simulink model "Masse_MultirotorSimHinf"  (R2018b)
settings: Solver=VariableStepAuto  StartTime=0.0  StopTime=Simulation.T_END  MaxStep=Simulation.TS_MAX  RelTol=1e-3  EnableMultiTasking=on
PreLoadFcn:
  | % InitializeParameters;
undefined symbols (not defined in the file): Aero, armed, ctrl_state, INIT_PARAM_VECTOR, Initial, K_i, K_p, Motor, mpc_att_sp, mpc_ctrl_state, mpc_manual, mpc_pos_sp_triplet, mpc_vehicle_land_detected, mpc_vehicle_status, Simulation, SOF1, SOF2, Uav, Upsilon, v_att_sp, v_control_mode
libraries: simulink_extras x9, simulink x6, dspstat3 x1, Px4Library x1
(part 3 of 11)

== system Masse_MultirotorSimHinf/Quadrotor Quaternion Model/Compute S Matrix2 ==
  quaternion : Inport
  MATLAB Function : MATLAB Function  TreatAsAtomicUnit=on
  rotationMatrix : Outport
  wires:
  quaternion/1 -> MATLAB Function/1(q)
  MATLAB Function/1(S) -> rotationMatrix/1

== system Masse_MultirotorSimHinf/Quadrotor Quaternion Model/Normalise Quaternion ==
  quaternion : Inport
  MATLAB Function : MATLAB Function  TreatAsAtomicUnit=on
  normalised : Outport
  wires:
  quaternion/1 -> MATLAB Function/1(q)
  MATLAB Function/1(qOut) -> normalised/1

== system Masse_MultirotorSimHinf/Quadrotor Quaternion Model/Quaternion to Euler Angles ==
  quaternion : Inport
  MATLAB Function : MATLAB Function  TreatAsAtomicUnit=on
  euler : Outport
  wires:
  quaternion/1 -> MATLAB Function/1(quat)
  MATLAB Function/1(eul) -> euler/1

== system Masse_MultirotorSimHinf/Quadrotor Quaternion Model/Quaternion to Rotation Matrix ==
  quaternion : Inport
  MATLAB Function : MATLAB Function  TreatAsAtomicUnit=on
  rotationMatrix : Outport
  wires:
  MATLAB Function/1(R) -> rotationMatrix/1
  quaternion/1 -> MATLAB Function/1(q)

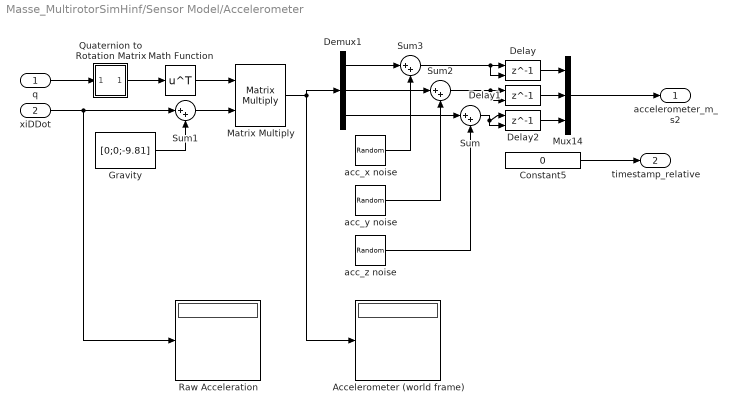
== system Masse_MultirotorSimHinf/Sensor Model/Accelerometer ==
  q : Inport
  xiDDot : Inport  Port=2  Unit=m/s^2
  Accelerometer (world frame) : Display
  Constant5 : Constant  Value=0
  Delay : Delay  DelayLength=1  InitialConditionSource=Input port  SampleTime=1/400
      settings: InputPortMap=u0,p4
  Delay1 : Delay  DelayLength=1  InitialConditionSource=Input port  SampleTime=1/400
      settings: InputPortMap=u0,p4
  Delay2 : Delay  DelayLength=1  InitialConditionSource=Input port  SampleTime=1/400
      settings: InputPortMap=u0,p4
  Demux1 : Demux  Outputs=3
  Gravity : Constant  Value=[0;0;-9.81]
  Math Function : Math  Operator=transpose  SaturateOnIntegerOverflow=on
  Matrix Multiply : Product  Multiplication=Matrix(*)
  Mux14 : Mux  Inputs=3
  Quaternion to Rotation Matrix : Subsystem  AncestorBlock=QuaternionLibrary/Quaternion to Rotation Matrix
      mask help: Convert an orientation quaternion to an orthogonal transformation matrix
      mask Help:
      | Convert an orientation quaternion
      | [q1 q2 q3 q4]
      | where:
      | - q1 is the rotation in radians
      | - [q2 q3 q4] is the vector around which the rotation is performed)
      | to an orthogonal transformation matrix
      | Based on code from the PX4 firmware: https://github.com/PX4/Firmware
      mask Display: disp('Q2R')
  Raw Acceleration : Display
  Sum{,1..3} (4 alike) : Sum  Inputs=|++
  acc_x noise : RandomNumber  Variance=0.012^2  SampleTime=1/400
  acc_y noise : RandomNumber  Variance=0.012^2  SampleTime=1/400
  acc_z noise : RandomNumber  Variance=0.02^2  SampleTime=1/400
  accelerometer_m_s2 : Outport  Unit=m/s^2  SampleTime=1/400
  timestamp_relative : Outport  Port=2  Unit=µs  SampleTime=1/400
  wires:
  Quaternion to Rotation Matrix/1(rotationMatrix) -> Math Function/1
  Math Function/1 -> Matrix Multiply/1
  Matrix Multiply/1 -> Accelerometer (world frame)/1, Demux1/1
  Gravity/1 -> Sum1/2
  Sum1/1 -> Matrix Multiply/2
  Mux14/1 -> accelerometer_m_s2/1
  xiDDot/1 -> Raw Acceleration/1, Sum1/1
  q/1 -> Quaternion to Rotation Matrix/1(quaternion)
  Constant5/1 -> timestamp_relative/1
  Demux1/1 -> Sum3/1
  Demux1/2 -> Sum2/1
  Demux1/3 -> Sum/1
  Sum/1 -> Delay2/2, Delay2/1
  acc_z noise/1 -> Sum/2
  Sum2/1 -> Delay1/2, Delay1/1
  Sum3/1 -> Delay/2, Delay/1
  acc_y noise/1 -> Sum2/2
  acc_x noise/1 -> Sum3/2
  Delay/1 -> Mux14/1
  Delay1/1 -> Mux14/2
  Delay2/1 -> Mux14/3

== system Masse_MultirotorSimHinf/Sensor Model/Barometer ==
  xi : Inport  Unit=m
  timestamp : Inport  Port=2  Unit=µs
  Add : Sum  Inputs=+-
  Scope : Scope
  Select altitude : Selector  InputPortWidth=3  IndexOptions=Index vector (dialog)  Indices=3  OutputSizes=1
  Sum : Sum  Inputs=|++
  To 400 Hz : RateTransition  Deterministic=off  OutPortSampleTime=1/250
  To 400 Hz1 : RateTransition  OutPortSampleTime=1/400
  To 50 Hz : RateTransition  OutPortSampleTime=1/50
  To 50 Hz1 : RateTransition  OutPortSampleTime=1/50
  barro noise : RandomNumber  Variance=1/3^2  SampleTime=0.01
  baro_alt_meter : Outport  Unit=m  SampleTime=1/400
  timestamp_relative : Outport  Port=2  Unit=µs
  wires:
  barro noise/1 -> Sum/2
  Sum/1 -> To 50 Hz1/1
  xi/1 -> Select altitude/1
  Select altitude/1 -> Sum/1
  Add/1 -> timestamp_relative/1, Scope/1
  To 400 Hz1/1 -> Add/2
  To 50 Hz/1 -> To 400 Hz/1
  To 400 Hz/1 -> Add/1
  timestamp/1 -> To 50 Hz/1, To 400 Hz1/1
  To 50 Hz1/1 -> baro_alt_meter/1

== system Masse_MultirotorSimHinf/Sensor Model/Global reprojection ==
  x : Inport
  y : Inport  Port=2
  map_projection_reproject : MATLAB Function  TreatAsAtomicUnit=on
  lat : Outport
  lon : Outport  Port=2
  wires:
  y/1 -> map_projection_reproject/2(y)
  map_projection_reproject/2(lon) -> lon/1
  x/1 -> map_projection_reproject/1(x)
  map_projection_reproject/1(lat) -> lat/1

== system Masse_MultirotorSimHinf/Sensor Model/Gyroscope ==
  nuBody : Inport  Unit=rad/s
  Bias : Constant  Commented=on  Value=[0.0001;0.0001;0.0001]
  Delay1 : Delay  DelayLength=1  InitialConditionSource=Input port  SampleTime=1/400
      settings: InputPortMap=u0,p4
  Delay2 : Delay  DelayLength=1  InitialConditionSource=Input port  SampleTime=1/400
      settings: InputPortMap=u0,p4
  Delay4 : Delay  DelayLength=1  InitialConditionSource=Input port  SampleTime=1/400
      settings: InputPortMap=u0,p4
  Demux : Demux  Outputs=3
  Mux : Mux  Inputs=3
  Sum2 : Sum  Inputs=++|
  gyro_rad : Outport  Unit=rad/s  SampleTime=1/400
  wires:
  Sum2/1 -> Demux/1
  Mux/1 -> gyro_rad/1
  Bias/1 -> Sum2/1
  nuBody/1 -> Sum2/2
  Delay4/1 -> Mux/2
  Delay2/1 -> Mux/3
  Delay1/1 -> Mux/1
  Demux/1 -> Delay1/2, Delay1/1
  Demux/2 -> Delay4/2, Delay4/1
  Demux/3 -> Delay2/2, Delay2/1

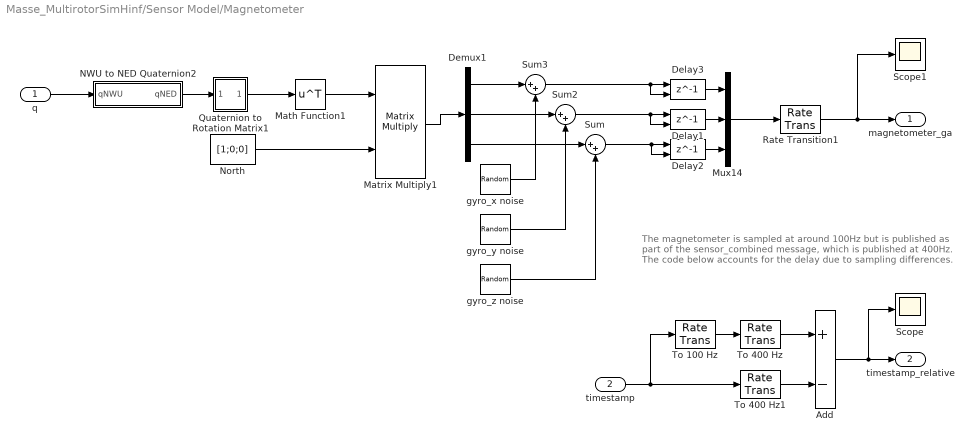
== system Masse_MultirotorSimHinf/Sensor Model/Magnetometer ==
  note: The magnetometer is sampled at around 100Hz but is published
      | as part of the sensor_combined message, which is published at
      | 400Hz. The code below accounts for the delay due to sampling
      | differences.
  q : Inport
  timestamp : Inport  Port=2
  Add : Sum  Inputs=+-
  Delay1 : Delay  DelayLength=1  InitialConditionSource=Input port  SampleTime=1/100
      settings: InputPortMap=u0,p4
  Delay2 : Delay  DelayLength=1  InitialConditionSource=Input port  SampleTime=1/100
      settings: InputPortMap=u0,p4
  Delay3 : Delay  DelayLength=1  InitialConditionSource=Input port  SampleTime=1/100
      settings: InputPortMap=u0,p4
  Demux1 : Demux  Outputs=3
  Math Function1 : Math  Operator=transpose  SaturateOnIntegerOverflow=on
  Matrix Multiply1 : Product  Multiplication=Matrix(*)
  Mux14 : Mux  Inputs=3
  NWU to NED Quaternion2 : Subsystem  AncestorBlock=Px4Library/NWU to NED Quaternion  mask(Coordinate transform){}
      mask help:
      | Convert a 3x1 vector or 4x1 quaternion from a North West Up to a North East Down coordinate system.
      |
      | The appropriate coordinate transform is automatically selected based on the input size.
  North : Constant  Value=[1;0;0]
  Quaternion to Rotation Matrix1 : Subsystem  AncestorBlock=QuaternionLibrary/Quaternion to Rotation Matrix
      mask help: Convert an orientation quaternion to an orthogonal transformation matrix
      mask Help:
      | Convert an orientation quaternion
      | [q1 q2 q3 q4]
      | where:
      | - q1 is the rotation in radians
      | - [q2 q3 q4] is the vector around which the rotation is performed)
      | to an orthogonal transformation matrix
      | Based on code from the PX4 firmware: https://github.com/PX4/Firmware
      mask Display: disp('Q2R')
  Rate Transition1 : RateTransition  Deterministic=off  OutPortSampleTime=1/100
  Scope : Scope
  Scope1 : Scope
  Sum : Sum  Inputs=|++
  Sum2 : Sum  Inputs=|++
  Sum3 : Sum  Inputs=|++
  To 100 Hz : RateTransition  OutPortSampleTime=1/100
  To 400 Hz : RateTransition  Deterministic=off  OutPortSampleTime=1/250
  To 400 Hz1 : RateTransition  OutPortSampleTime=1/400
  gyro_x noise : RandomNumber  Variance=0.001^2  SampleTime=1/400
  gyro_y noise : RandomNumber  Variance=0.001^2  SampleTime=1/400
  gyro_z noise : RandomNumber  Variance=0.001^2  SampleTime=1/400
  magnetometer_ga : Outport  Unit=G  SampleTime=1/250
  timestamp_relative : Outport  Port=2  Unit=µs  SampleTime=1/250
  wires:
  NWU to NED Quaternion2/1(qNED) -> Quaternion to Rotation Matrix1/1(quaternion)
  Quaternion to Rotation Matrix1/1(rotationMatrix) -> Math Function1/1
  q/1 -> NWU to NED Quaternion2/1(qNWU)
  North/1 -> Matrix Multiply1/2
  Math Function1/1 -> Matrix Multiply1/1
  Add/1 -> timestamp_relative/1, Scope/1
  Matrix Multiply1/1 -> Demux1/1
  Demux1/1 -> Sum3/1
  Demux1/2 -> Sum2/1
  Demux1/3 -> Sum/1
  Sum/1 -> Delay2/2, Delay2/1
  gyro_z noise/1 -> Sum/2
  Sum2/1 -> Delay1/2, Delay1/1
  gyro_y noise/1 -> Sum2/2
  gyro_x noise/1 -> Sum3/2
  Mux14/1 -> Rate Transition1/1
  To 400 Hz1/1 -> Add/2
  To 100 Hz/1 -> To 400 Hz/1
  To 400 Hz/1 -> Add/1
  Rate Transition1/1 -> Scope1/1, magnetometer_ga/1
  timestamp/1 -> To 100 Hz/1, To 400 Hz1/1
  Delay3/1 -> Mux14/1
  Sum3/1 -> Delay3/2, Delay3/1
  Delay1/1 -> Mux14/2
  Delay2/1 -> Mux14/3

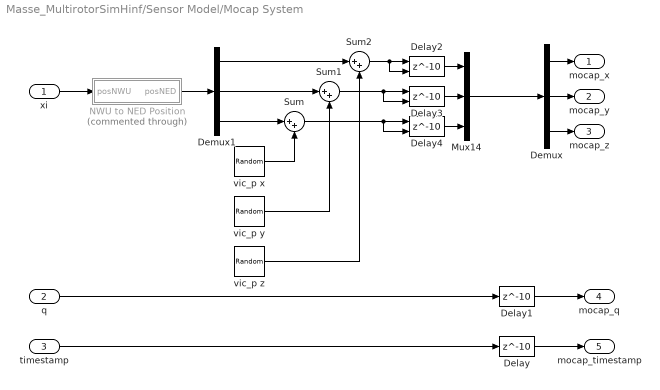
== system Masse_MultirotorSimHinf/Sensor Model/Mocap System ==
  xi : Inport
  q : Inport  Port=2
  timestamp : Inport  Port=3
  Delay : Delay  DelayLength=10  SampleTime=1/100
  Delay1 : Delay  DelayLength=10  SampleTime=1/100
  Delay2 : Delay  DelayLength=10  InitialConditionSource=Input port  SampleTime=1/100
      settings: InputPortMap=u0,p4
  Delay3 : Delay  DelayLength=10  InitialConditionSource=Input port  SampleTime=1/100
      settings: InputPortMap=u0,p4
  Delay4 : Delay  DelayLength=10  InitialConditionSource=Input port  SampleTime=1/100
      settings: InputPortMap=u0,p4
  Demux : Demux  Outputs=3
  Demux1 : Demux  Outputs=3
  Mux14 : Mux  Inputs=3
  NWU to NED Position : Subsystem  Commented=through  AncestorBlock=Px4Library/NWU to NED Position  mask(Coordinate transform){}
      mask help:
      | Convert a 3x1 vector or 4x1 quaternion from a North West Up to a North East Down coordinate system.
      |
      | The appropriate coordinate transform is automatically selected based on the input size.
  Sum : Sum  Inputs=|++
  Sum1 : Sum  Inputs=|++
  Sum2 : Sum  Inputs=|++
  vic_p x : RandomNumber  Variance=0.001^2  SampleTime=0.01
  vic_p y : RandomNumber  Variance=0.001^2  SampleTime=0.01
  vic_p z : RandomNumber  Variance=0.001^2  SampleTime=0.01
  mocap_x : Outport
  mocap_y : Outport  Port=2
  mocap_z : Outport  Port=3
  mocap_q : Outport  Port=4
  mocap_timestamp : Outport  Port=5
  wires:
  q/1 -> Delay1/1
  timestamp/1 -> Delay/1
  Delay/1 -> mocap_timestamp/1
  Delay1/1 -> mocap_q/1
  Demux1/1 -> Sum2/1
  Demux1/2 -> Sum1/1
  NWU to NED Position/1(posNED) -> Demux1/1
  Demux1/3 -> Sum/1
  Sum/1 -> Delay4/2, Delay4/1
  vic_p x/1 -> Sum/2
  Sum1/1 -> Delay3/2, Delay3/1
  Sum2/1 -> Delay2/2, Delay2/1
  vic_p y/1 -> Sum1/2
  vic_p z/1 -> Sum2/2
  xi/1 -> NWU to NED Position/1(posNWU)
  Demux/3 -> mocap_z/1
  Demux/2 -> mocap_y/1
  Demux/1 -> mocap_x/1
  Mux14/1 -> Demux/1
  Delay2/1 -> Mux14/1
  Delay3/1 -> Mux14/2
  Delay4/1 -> Mux14/3

== system Masse_MultirotorSimHinf/Sensor Model/NWU to NED Position3 ==
  posNWU : Inport
  Multiply : Product  Inputs=**
  Position gain : Constant  Value=[1; -1; -1]
  posNED : Outport
  wires:
  posNWU/1 -> Multiply/1
  Multiply/1 -> posNED/1
  Position gain/1 -> Multiply/2

== system Masse_MultirotorSimHinf/Sensor Model/Quaternion to Euler Angles ==
  quaternion : Inport
  MATLAB Function : MATLAB Function  TreatAsAtomicUnit=on
  euler : Outport
  wires:
  quaternion/1 -> MATLAB Function/1(quat)
  MATLAB Function/1(eul) -> euler/1

== system Masse_MultirotorSimHinf/Sensor Model/Quaternion to Euler Angles1 ==
  quaternion : Inport
  MATLAB Function : MATLAB Function  TreatAsAtomicUnit=on
  euler : Outport
  wires:
  quaternion/1 -> MATLAB Function/1(quat)
  MATLAB Function/1(eul) -> euler/1

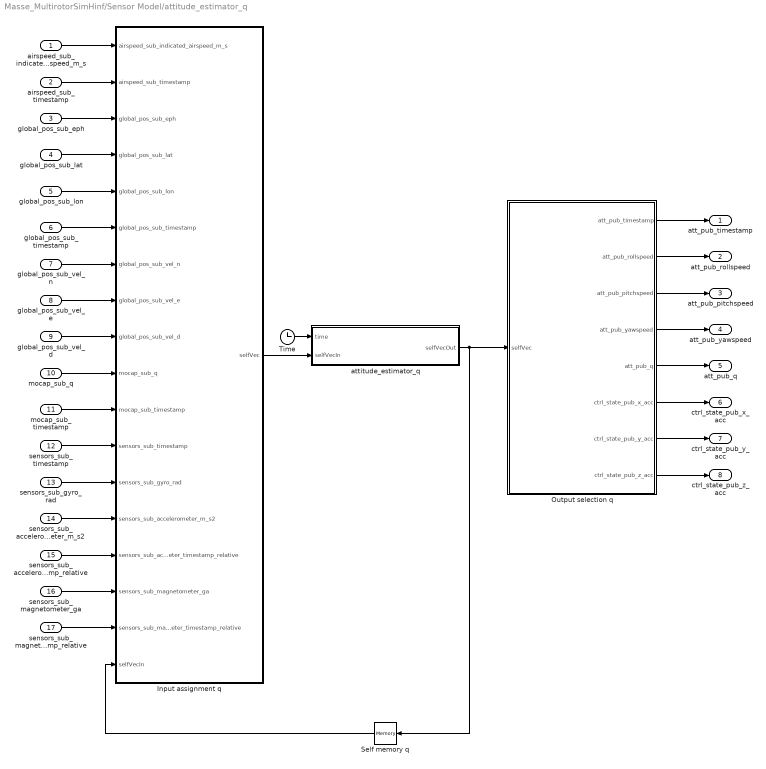
== system Masse_MultirotorSimHinf/Sensor Model/attitude_estimator_q ==
  airspeed_sub_indicated_airspeed_m_s : Inport
  airspeed_sub_timestamp : Inport  Port=2
  global_pos_sub_eph : Inport  Port=3
  global_pos_sub_lat : Inport  Port=4
  global_pos_sub_lon : Inport  Port=5
  global_pos_sub_timestamp : Inport  Port=6
  global_pos_sub_vel_n : Inport  Port=7
  global_pos_sub_vel_e : Inport  Port=8
  global_pos_sub_vel_d : Inport  Port=9
  mocap_sub_q : Inport  Port=10
  mocap_sub_timestamp : Inport  Port=11
  sensors_sub_timestamp : Inport  Port=12
  sensors_sub_gyro_rad : Inport  Port=13
  sensors_sub_accelerometer_m_s2 : Inport  Port=14
  sensors_sub_accelerometer_timestamp_relative : Inport  Port=15
  sensors_sub_magnetometer_ga : Inport  Port=16
  sensors_sub_magnetometer_timestamp_relative : Inport  Port=17
  Input assignment q : MATLAB Function  TreatAsAtomicUnit=on
  Output selection q : MATLAB Function  TreatAsAtomicUnit=on
  Self memory q : Memory  InitialCondition=[ATT_ACC_COMP, 0, 0, 0, 0, 0, 0, 0, FW_ARSP_MODE, 0, 0, 0, 0, 0, 0, 0, 0, INIT_Q(1), INIT_Q(2), INIT_Q(3), INIT_Q(4), ATT_BIAS_MAX, 0, 0, INIT_Q(1), INIT_Q(2), INIT_Q(3), INIT_Q(4), 0, 0, 0, 0, 0, 0, 0, 0, 0, 0, 0, 0, 0.02, 0, ATT_EXT_HDG_M, 0, 0, 0, 0, 0, 0, 0, 0, 0, 0, 0, 0, 0, 0, 0, 0, 0, 0, 0, 0, 0, 0, 0, 0, 0, 0, 0, 0, 0, 0, 0, 0, 0, 0, 0, 0, 0, 0, 0, 0, 0, 0, 0, 0, 0, 0, 0, 0, 0, 0, 0, 0, 0, 0, 0, 0, 0, 0, 0, 0, 0, 0, 0, 0, 0, 0, 0, 0, 0, 0, 0, 0, 0, 0, 0, 0, 0, 0, 0, 0, 0, 0, 0, 0, 0, 0, 0, 0, 0, ATT_MAG_DECL, ATT_MAG_DECL_A, 0, 0, 0, 0, 0, 0, 0, 0, 0, 0, 0, 0, 0, 0, 0, 0, 0, 0, 0, 0, 0, 0, INIT_Q(1), INIT_Q(2), INIT_Q(3), INIT_Q(4), 0, 0, 0, 0, 0, 0, 0, 0, 0, 0, 0, 0, 0, 0, 0, 0, 0, 0, 0, 0, 0, 0, 0, 0, 0, 0, 0, 0, 0, 0, 0, 0, 0, 0, 0, 0, 0, 0, 0, ATT_W_ACC, ATT_W_EXT_HDG, ATT_W_GYRO_BIAS, ATT_W_MAG, 0, 0]
  Time : Clock
  attitude_estimator_q : MATLAB Function  TreatAsAtomicUnit=on  SystemSampleTime=Q_SAMPLING_PERIOD
  att_pub_timestamp : Outport
  att_pub_rollspeed : Outport  Port=2
  att_pub_pitchspeed : Outport  Port=3
  att_pub_yawspeed : Outport  Port=4
  att_pub_q : Outport  Port=5
  ctrl_state_pub_x_acc : Outport  Port=6
  ctrl_state_pub_y_acc : Outport  Port=7
  ctrl_state_pub_z_acc : Outport  Port=8
  wires:
  Output selection q/8(ctrl_state_pub_z_acc) -> ctrl_state_pub_z_acc/1
  Output selection q/7(ctrl_state_pub_y_acc) -> ctrl_state_pub_y_acc/1
  Output selection q/6(ctrl_state_pub_x_acc) -> ctrl_state_pub_x_acc/1
  Output selection q/5(att_pub_q) -> att_pub_q/1
  Output selection q/4(att_pub_yawspeed) -> att_pub_yawspeed/1
  Output selection q/3(att_pub_pitchspeed) -> att_pub_pitchspeed/1
  Output selection q/2(att_pub_rollspeed) -> att_pub_rollspeed/1
  Output selection q/1(att_pub_timestamp) -> att_pub_timestamp/1
  sensors_sub_magnetometer_timestamp_relative/1 -> Input assignment q/17(sensors_sub_magnetometer_timestamp_relative)
  sensors_sub_magnetometer_ga/1 -> Input assignment q/16(sensors_sub_magnetometer_ga)
  sensors_sub_accelerometer_timestamp_relative/1 -> Input assignment q/15(sensors_sub_accelerometer_timestamp_relative)
  sensors_sub_accelerometer_m_s2/1 -> Input assignment q/14(sensors_sub_accelerometer_m_s2)
  sensors_sub_gyro_rad/1 -> Input assignment q/13(sensors_sub_gyro_rad)
  sensors_sub_timestamp/1 -> Input assignment q/12(sensors_sub_timestamp)
  mocap_sub_timestamp/1 -> Input assignment q/11(mocap_sub_timestamp)
  mocap_sub_q/1 -> Input assignment q/10(mocap_sub_q)
  global_pos_sub_vel_d/1 -> Input assignment q/9(global_pos_sub_vel_d)
  global_pos_sub_vel_e/1 -> Input assignment q/8(global_pos_sub_vel_e)
  global_pos_sub_vel_n/1 -> Input assignment q/7(global_pos_sub_vel_n)
  global_pos_sub_timestamp/1 -> Input assignment q/6(global_pos_sub_timestamp)
  global_pos_sub_lon/1 -> Input assignment q/5(global_pos_sub_lon)
  global_pos_sub_lat/1 -> Input assignment q/4(global_pos_sub_lat)
  global_pos_sub_eph/1 -> Input assignment q/3(global_pos_sub_eph)
  airspeed_sub_timestamp/1 -> Input assignment q/2(airspeed_sub_timestamp)
  airspeed_sub_indicated_airspeed_m_s/1 -> Input assignment q/1(airspeed_sub_indicated_airspeed_m_s)
  Time/1 -> attitude_estimator_q/1(time)
  Self memory q/1 -> Input assignment q/18(selfVecIn)
  attitude_estimator_q/1(selfVecOut) -> Self memory q/1, Output selection q/1(selfVec)
  Input assignment q/1(selfVec) -> attitude_estimator_q/2(selfVecIn)

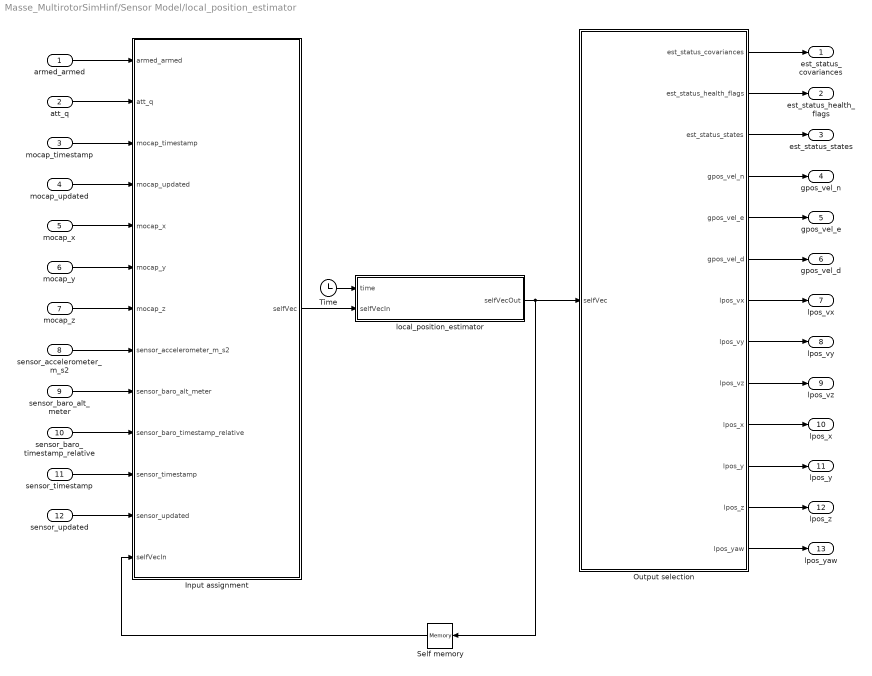
== system Masse_MultirotorSimHinf/Sensor Model/local_position_estimator ==
  armed_armed : Inport
  att_q : Inport  Port=2
  mocap_timestamp : Inport  Port=3
  mocap_updated : Inport  Port=4
  mocap_x : Inport  Port=5
  mocap_y : Inport  Port=6
  mocap_z : Inport  Port=7
  sensor_accelerometer_m_s2 : Inport  Port=8
  sensor_baro_alt_meter : Inport  Port=9
  sensor_baro_timestamp_relative : Inport  Port=10
  sensor_timestamp : Inport  Port=11
  sensor_updated : Inport  Port=12
  Input assignment : MATLAB Function  TreatAsAtomicUnit=on
  Output selection : MATLAB Function  TreatAsAtomicUnit=on
  Self memory : Memory  InitialCondition=[0, 0, 0, 0, 0, 0, 0, 0, 0, 0, 0, 0, 0, 0, 0, 0, 0, 0, 0, 0, 0, 0, 0, 0, 0, 0, 0, 0, 0, 0, 0, 0, 0, 0, 0, 0, 0, 0, 0, 0, 0, 0, 0, 0, 0, 0, 0, 0, 0, 0, 0, 0, 0, 0, 0, 0, 0, 0, 0, 0, 0, 0, 0, 0, 0, 0, 0, 0, 0, 0, 0, 0, 0, 0, 0, 0, 0, 0, 0, 0, 0, 0, 0, 0, 0, 0, 0, 0, 0, 0, 0, 0, 0, 0, 0, 0, 0, 0, 0, 0, 0, 0, 0, 0, 0, 0, 0, 0, 0, 0, 0, 0, 0, 0, 0, 0, 0, 0, 0, 0, 0, 0, 0, 0, 0, 0, 0, 0, 0, 0, 0, 8.82050518214, 12.094592431, 13.9876612368, 16.0875642296, 17.8797700658, 19.6465647819, 1e-1, 2.0, 2.0, 2.0, 2^2, 2^0, 2^1, 2^7, 2^1, 2^6, 2^0, 2^4, 2^5, 2^2, 2^3, 0, 10.0, 8, 0, 0, 0, 0, 0, 0, 0, 0, 0, 0, 8, 0, 0, 0, 0, 0, 0, 0, 0, 0, 0, 8, 0, 0, 0, 0, 0, 0, 0, 0, 0, 0, 2*LPE_VXY_PUB*LPE_VXY_PUB, 0, 0, 0, 0, 0, 0, 0, 0, 0, 0, 2*LPE_VXY_PUB*LPE_VXY_PUB, 0, 0, 0, 0, 0, 0, 0, 0, 0, 0, 2*LPE_VXY_PUB*LPE_VXY_PUB, 0, 0, 0, 0, 0, 0, 0, 0, 0, 0, 1e-6, 0, 0, 0, 0, 0, 0, 0, 0, 0, 0, 1e-6, 0, 0, 0, 0, 0, 0, 0, 0, 0, 0, 1e-6, 0, 0, 0, 0, 0, 0, 0, 0, 0, 0, 8, 1.0e6, 0, 0, 0, 0, 0, 0, 0, 0, 0, 0, 0, 0, 0, 0, 0, 0, 0, 0, 0, 0, 0, 0, 0, 0, 0, 0, 0, 0, 0, 0, 0, 0, 0, 0, 0, 0, 0, 0, 0, 0, 0, 0, 0, 0, 0, 0, 0, 0, 0, 0, 0, 0, 0, 0, 0, 0, 0, 0, 0, 0, 0, 0, 0, 0, 0, 0, 0, 0, 0, 0, 0, 0, 0, 0, 0, 0, 0, 0, 0, 0, 0, 0, 0, 0, 0, 0, 0, 0, 0, 0, 0, 0, 0, 0, 0, 0, 0, 0, 0, 0, 0, 0, 0, 0, 0, 0, 0, 0, 0, 0, 0, 0, 0, 0, 0, 0, 0, 0, 2^0, 2^3, 2^1, 2^7, 2^2, 2^6, 2^4, 2^5, 0, LPE_ACC_XY, 0, LPE_ACC_Z, LPE_SAMPLING_PERIOD, LPE_X_LP, 0, 0, 0, 0, 0, 0, LPE_BAR_Z, LPE_SAMPLING_PERIOD, 0, 0, 0, 0, LPE_FAKE_ORIGIN, 0, LPE_FGYRO_HP, LPE_FGYRO_HP, LPE_FLW_QMIN, LPE_FLW_R, LPE_FLW_RR, LPE_FLW_SCALE, LPE_FLW_OFF_Z, LPE_FUSION, 0, LPE_GPS_DELAY, LPE_EPH_MAX, LPE_EPV_MAX, LPE_GPS_VXY, LPE_GPS_VZ, LPE_GPS_XY, LPE_GPS_Z, LPE_LAT, LPE_LON, 0, 0, LPE_LAND_VXY, LPE_LAND_Z, 0, LPE_LDR_OFF_Z, LPE_LDR_Z, 0, 0, 0, 0, 0, 0, 0, LPE_VIC_P, LPE_PN_B, LPE_PN_P, LPE_PN_T, LPE_PN_V, 8, 0, 0, 0, 0, 0, 0, 0, 0, 0, 0, 0, 0, 0, 0, 0, 0, 0, 0, 0, 0, 0, 0, 0, 0, 0, 0, 0, 0, 0, 0, 0, 0, 0, 0, 0, 0, 0, 0, 0, 0, 0, 0, 0, 0, 0, 0, 0, 0, 0, 0, 0, 0, 0, 0, 0, 0, 0, 0, 0, 0, 0, 0, 0, 0, 0, 0, 0, 0, 0, 0, 0, 0, 0, 0, 255, 0, LPE_SNR_OFF_Z, LPE_SNR_Z, 0, 0, 0, 0, 0, 0, 0, 0, 0, 0, 0, 0, 0, 0, 0, 0, 0, 0, 0, 0, 0, 0, 0, 0, 0, 0, 0, 0, 0, 0, 0, 0, 0, 0, 0, 0, 0, 0, 0, 1, 1, LPE_T_MAX_GRADE, 0, 0, 0, 0, 0, 0, 0, 0, 0, 0, 0, LPE_VIS_DELAY, LPE_VIS_XY, LPE_VIS_Z, LPE_VXY_PUB, 0, 0, 0, 0, 0, 0, 0, 0, 0, 0, 0, 0, 0, 0, 0, 0, 0, 0, 0, 0, 0, 0, 0, 0, 0, 0, 0, 0, 0, 0, 0, 0, 0, 0, 0, 0, 0, 0, 0, 0, 0, 0, 0, 0, 0, 0, 0, 0, 0, 0, 0, 0, 0, 0, 0, 0, 0, 0, 0, 0, 0, 0, 0, 0, 0, 0, 0, 0, 0, 0, 0, 0, 0, 0, 0, 0, 0, 0, 0, 0, 0, 0, 0, 0, 0, 0, 0, 0, 0, 0, 0, 0, 0, 0, 0, 0, 0, 0, 0, 0, 0, 0, 0, 0, 0, 0, 0, 0, 0, 0, 1, 1, LPE_SAMPLING_PERIOD, LPE_X_LP, 0, 0, 0, 0, 0, 0, 0, 0, 0, 0, LPE_Z_PUB]
  Time : Clock
  local_position_estimator : MATLAB Function  TreatAsAtomicUnit=on  SystemSampleTime=LPE_SAMPLING_PERIOD
  est_status_covariances : Outport
  est_status_health_flags : Outport  Port=2
  est_status_states : Outport  Port=3
  gpos_vel_n : Outport  Port=4
  gpos_vel_e : Outport  Port=5
  gpos_vel_d : Outport  Port=6
  lpos_vx : Outport  Port=7
  lpos_vy : Outport  Port=8
  lpos_vz : Outport  Port=9
  lpos_x : Outport  Port=10
  lpos_y : Outport  Port=11
  lpos_z : Outport  Port=12
  lpos_yaw : Outport  Port=13
  wires:
  Output selection/13(lpos_yaw) -> lpos_yaw/1
  Output selection/12(lpos_z) -> lpos_z/1
  Output selection/11(lpos_y) -> lpos_y/1
  Output selection/10(lpos_x) -> lpos_x/1
  Output selection/9(lpos_vz) -> lpos_vz/1
  Output selection/8(lpos_vy) -> lpos_vy/1
  Output selection/7(lpos_vx) -> lpos_vx/1
  Output selection/6(gpos_vel_d) -> gpos_vel_d/1
  Output selection/5(gpos_vel_e) -> gpos_vel_e/1
  Output selection/4(gpos_vel_n) -> gpos_vel_n/1
  Output selection/3(est_status_states) -> est_status_states/1
  Output selection/2(est_status_health_flags) -> est_status_health_flags/1
  Output selection/1(est_status_covariances) -> est_status_covariances/1
  sensor_updated/1 -> Input assignment/12(sensor_updated)
  sensor_timestamp/1 -> Input assignment/11(sensor_timestamp)
  sensor_baro_timestamp_relative/1 -> Input assignment/10(sensor_baro_timestamp_relative)
  sensor_baro_alt_meter/1 -> Input assignment/9(sensor_baro_alt_meter)
  sensor_accelerometer_m_s2/1 -> Input assignment/8(sensor_accelerometer_m_s2)
  mocap_z/1 -> Input assignment/7(mocap_z)
  mocap_y/1 -> Input assignment/6(mocap_y)
  mocap_x/1 -> Input assignment/5(mocap_x)
  mocap_updated/1 -> Input assignment/4(mocap_updated)
  mocap_timestamp/1 -> Input assignment/3(mocap_timestamp)
  att_q/1 -> Input assignment/2(att_q)
  armed_armed/1 -> Input assignment/1(armed_armed)
  Time/1 -> local_position_estimator/1(time)
  Self memory/1 -> Input assignment/13(selfVecIn)
  local_position_estimator/1(selfVecOut) -> Self memory/1, Output selection/1(selfVec)
  Input assignment/1(selfVec) -> local_position_estimator/2(selfVecIn)

== system Masse_MultirotorSimHinf/att_mixerInput/Euler Angles to Quaternion ==
  euler : Inport
  MATLAB Function : MATLAB Function  TreatAsAtomicUnit=on
  quaternion : Outport
  wires:
  MATLAB Function/1(quat) -> quaternion/1
  euler/1 -> MATLAB Function/1(eulerAngles)

== system Masse_MultirotorSimHinf/att_mixerInput/Quaternion to Euler Angles2 ==
  quaternion : Inport
  MATLAB Function : MATLAB Function  TreatAsAtomicUnit=on
  euler : Outport
  wires:
  quaternion/1 -> MATLAB Function/1(quat)
  MATLAB Function/1(eul) -> euler/1

== system Masse_MultirotorSimHinf/att_mixerInput/Quaternion to Euler Angles3 ==
  quaternion : Inport
  MATLAB Function : MATLAB Function  TreatAsAtomicUnit=on
  euler : Outport
  wires:
  quaternion/1 -> MATLAB Function/1(quat)
  MATLAB Function/1(eul) -> euler/1

== system Masse_MultirotorSimHinf/mc_att_control/Flags ==
  armed : Inport
  control_attitude : Inport  Port=2
  control_auto : Inport  Port=3
  control_manual : Inport  Port=4
  control_rates : Inport  Port=5
  control_velocity : Inport  Port=6
  BusIn : Inport  Port=7
  Flags bus assignment : BusAssignment  AssignedSignals=armed.armed,v_control_mode.flag_control_attitude_enabled,v_control_mode.flag_control_auto_enabled,v_control_mode.flag_control_manual_enabled,v_control_mode.flag_control_rates_enabled,v_control_mode.flag_control_velocity_enabled
  Bus : Outport
  wires:
  control_rates/1 -> Flags bus assignment/6
  control_manual/1 -> Flags bus assignment/5
  control_attitude/1 -> Flags bus assignment/3
  armed/1 -> Flags bus assignment/2
  control_velocity/1 -> Flags bus assignment/7
  control_auto/1 -> Flags bus assignment/4
  BusIn/1 -> Flags bus assignment/1
  Flags bus assignment/1 -> Bus/1

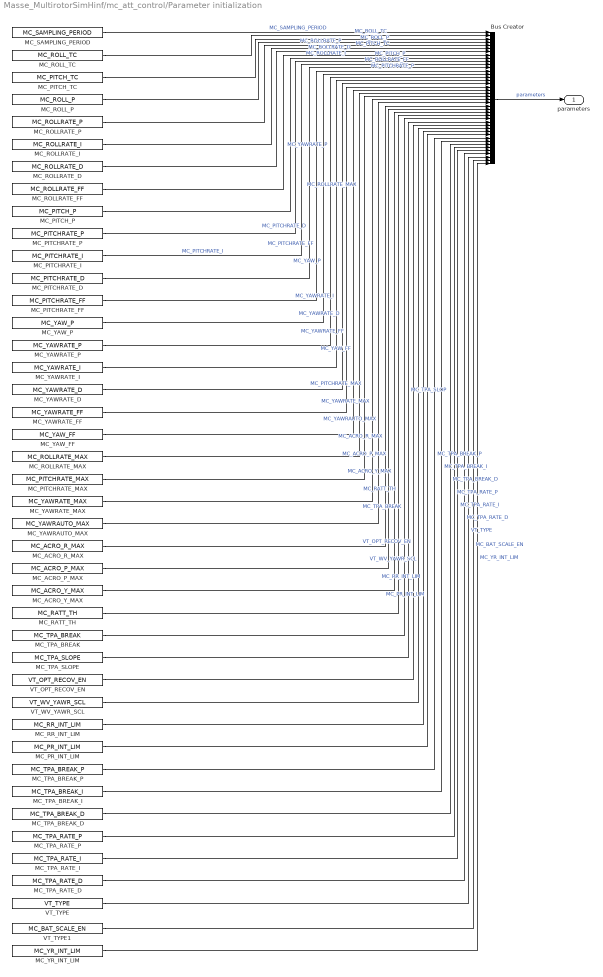
== system Masse_MultirotorSimHinf/mc_att_control/Parameter initialization ==
  Bus Creator : BusCreator  Inputs='MC_SAMPLING_PERIOD','MC_ROLL_TC','MC_PITCH_TC','MC_ROLL_P','MC_ROLLRATE_P','MC_ROLLRATE_I','MC_ROLLRATE_D','MC_ROLLRATE_FF','MC_PITCH_P','MC_PITCHRATE_P','MC_PITCHRATE_I','MC_PITCHRATE_D','MC_PITCHRATE_FF','MC_YAW_P','MC_YAWRATE_P','MC_YAWRATE_I','MC_YAWRATE_D','MC_YAWRATE_FF','MC_YAW_FF','MC_ROLLRATE_MAX','MC_PITCHRATE_MAX','MC_YAWRATE_MAX','MC_YAWRAUTO_MAX','MC_ACRO_R_MAX','MC_ACRO_P_MAX','MC_ACRO_Y_MAX','MC_RATT_TH','MC_TPA_BREAK','MC_TPA_SLOP','VT_OPT_RECOV_EN','VT_WV_YAWR_SCL','MC_RR_INT_LIM','MC_PR_INT_LIM','MC_TPA_BREAK_P','MC_TPA_BREAK_I','MC_TPA_BREAK_D','MC_TPA_RATE_P','MC_TPA_RATE_I','MC_TPA_RATE_D','VT_TYPE','MC_BAT_SCALE_EN','MC_YR_INT_LIM'  OutDataTypeStr=Bus: parameterBus
  MC_ACRO_P_MAX : Constant  Value=MC_ACRO_P_MAX
  MC_ACRO_R_MAX : Constant  Value=MC_ACRO_R_MAX
  MC_ACRO_Y_MAX : Constant  Value=MC_ACRO_Y_MAX
  MC_PITCHRATE_D : Constant  Value=MC_PITCHRATE_D
  MC_PITCHRATE_FF : Constant  Value=MC_PITCHRATE_FF
  MC_PITCHRATE_I : Constant  Value=MC_PITCHRATE_I
  MC_PITCHRATE_MAX : Constant  Value=MC_PITCHRATE_MAX
  MC_PITCHRATE_P : Constant  Value=MC_PITCHRATE_P
  MC_PITCH_P : Constant  Value=MC_PITCH_P
  MC_PITCH_TC : Constant  Value=MC_PITCH_TC
  MC_PR_INT_LIM : Constant  Value=MC_PR_INT_LIM
  MC_RATT_TH : Constant  Value=MC_RATT_TH
  MC_ROLLRATE_D : Constant  Value=MC_ROLLRATE_D
  MC_ROLLRATE_FF : Constant  Value=MC_ROLLRATE_FF
  MC_ROLLRATE_I : Constant  Value=MC_ROLLRATE_I
  MC_ROLLRATE_MAX : Constant  Value=MC_ROLLRATE_MAX
  MC_ROLLRATE_P : Constant  Value=MC_ROLLRATE_P
  MC_ROLL_P : Constant  Value=MC_ROLL_P
  MC_ROLL_TC : Constant  Value=MC_ROLL_TC
  MC_RR_INT_LIM : Constant  Value=MC_RR_INT_LIM
  MC_SAMPLING_PERIOD : Constant  Value=MC_SAMPLING_PERIOD
  MC_TPA_BREAK : Constant  Value=MC_TPA_BREAK
  MC_TPA_BREAK_D : Constant  Value=MC_TPA_BREAK_D
  MC_TPA_BREAK_I : Constant  Value=MC_TPA_BREAK_I
  MC_TPA_BREAK_P : Constant  Value=MC_TPA_BREAK_P
  MC_TPA_RATE_D : Constant  Value=MC_TPA_RATE_D
  MC_TPA_RATE_I : Constant  Value=MC_TPA_RATE_I
  MC_TPA_RATE_P : Constant  Value=MC_TPA_RATE_P
  MC_TPA_SLOPE : Constant  Value=MC_TPA_SLOPE
  MC_YAWRATE_D : Constant  Value=MC_YAWRATE_D
  MC_YAWRATE_FF : Constant  Value=MC_YAWRATE_FF
  MC_YAWRATE_I : Constant  Value=MC_YAWRATE_I
  MC_YAWRATE_MAX : Constant  Value=MC_YAWRATE_MAX
  MC_YAWRATE_P : Constant  Value=MC_YAWRATE_P
  MC_YAWRAUTO_MAX : Constant  Value=MC_YAWRAUTO_MAX
  MC_YAW_FF : Constant  Value=MC_YAW_FF
  MC_YAW_P : Constant  Value=MC_YAW_P
  MC_YR_INT_LIM : Constant  Value=MC_YR_INT_LIM
  VT_OPT_RECOV_EN : Constant  Value=VT_OPT_RECOV_EN
  VT_TYPE : Constant  Value=VT_TYPE
  VT_TYPE1 : Constant  Value=MC_BAT_SCALE_EN
  VT_WV_YAWR_SCL : Constant  Value=VT_WV_YAWR_SCL
  parameters : Outport
  wires:
  MC_RR_INT_LIM/1 -> Bus Creator/32  "MC_RR_INT_LIM"
  VT_TYPE1/1 -> Bus Creator/41  "MC_BAT_SCALE_EN"
  MC_TPA_BREAK_D/1 -> Bus Creator/36  "MC_TPA_BREAK_D"
  MC_TPA_BREAK_I/1 -> Bus Creator/35  "MC_TPA_BREAK_I"
  MC_TPA_BREAK_P/1 -> Bus Creator/34  "MC_TPA_BREAK_P"
  MC_YR_INT_LIM/1 -> Bus Creator/42  "MC_YR_INT_LIM"
  MC_TPA_RATE_D/1 -> Bus Creator/39  "MC_TPA_RATE_D"
  VT_TYPE/1 -> Bus Creator/40  "VT_TYPE"
  MC_TPA_BREAK/1 -> Bus Creator/28  "MC_TPA_BREAK"
  VT_WV_YAWR_SCL/1 -> Bus Creator/31  "VT_WV_YAWR_SCL"
  MC_TPA_SLOPE/1 -> Bus Creator/29  "MC_TPA_SLOP"
  MC_ACRO_R_MAX/1 -> Bus Creator/24  "MC_ACRO_R_MAX"
  Bus Creator/1 -> parameters/1  "parameters"
  MC_ACRO_P_MAX/1 -> Bus Creator/25  "MC_ACRO_P_MAX"
  MC_ACRO_Y_MAX/1 -> Bus Creator/26  "MC_ACRO_Y_MAX"
  VT_OPT_RECOV_EN/1 -> Bus Creator/30  "VT_OPT_RECOV_EN"
  MC_RATT_TH/1 -> Bus Creator/27  "MC_RATT_TH"
  MC_YAWRATE_MAX/1 -> Bus Creator/22  "MC_YAWRATE_MAX"
  MC_YAWRAUTO_MAX/1 -> Bus Creator/23  "MC_YAWRAUTO_MAX"
  MC_YAWRATE_P/1 -> Bus Creator/15  "MC_YAWRATE_P"
  MC_ROLL_TC/1 -> Bus Creator/2  "MC_ROLL_TC"
  MC_PITCH_P/1 -> Bus Creator/9  "MC_PITCH_P"
  MC_PITCH_TC/1 -> Bus Creator/3  "MC_PITCH_TC"
  MC_SAMPLING_PERIOD/1 -> Bus Creator/1  "MC_SAMPLING_PERIOD"
  MC_PITCHRATE_MAX/1 -> Bus Creator/21  "MC_PITCHRATE_MAX"
  MC_YAWRATE_I/1 -> Bus Creator/16  "MC_YAWRATE_I"
  MC_ROLL_P/1 -> Bus Creator/4  "MC_ROLL_P"
  MC_ROLLRATE_MAX/1 -> Bus Creator/20  "MC_ROLLRATE_MAX"
  MC_YAW_P/1 -> Bus Creator/14  "MC_YAW_P"
  MC_YAWRATE_FF/1 -> Bus Creator/18  "MC_YAWRATE_FF"
  MC_ROLLRATE_FF/1 -> Bus Creator/8  "MC_ROLLRATE_FF"
  MC_PITCHRATE_D/1 -> Bus Creator/12  "MC_PITCHRATE_D"
  MC_PITCHRATE_I/1 -> Bus Creator/11  "MC_PITCHRATE_I"
  MC_ROLLRATE_D/1 -> Bus Creator/7  "MC_ROLLRATE_D"
  MC_ROLLRATE_P/1 -> Bus Creator/5  "MC_ROLLRATE_P"
  MC_PITCHRATE_P/1 -> Bus Creator/10  "MC_PITCHRATE_P"
  MC_PITCHRATE_FF/1 -> Bus Creator/13  "MC_PITCHRATE_FF"
  MC_YAW_FF/1 -> Bus Creator/19  "MC_YAW_FF"
  MC_YAWRATE_D/1 -> Bus Creator/17  "MC_YAWRATE_D"
  MC_ROLLRATE_I/1 -> Bus Creator/6  "MC_ROLLRATE_I"
  MC_PR_INT_LIM/1 -> Bus Creator/33  "MC_PR_INT_LIM"
  MC_TPA_RATE_P/1 -> Bus Creator/37  "MC_TPA_RATE_P"
  MC_TPA_RATE_I/1 -> Bus Creator/38  "MC_TPA_RATE_I"

== system Masse_MultirotorSimHinf/Sensor Model/Accelerometer/Quaternion to Rotation Matrix ==
  quaternion : Inport
  MATLAB Function : MATLAB Function  TreatAsAtomicUnit=on
  rotationMatrix : Outport
  wires:
  MATLAB Function/1(R) -> rotationMatrix/1
  quaternion/1 -> MATLAB Function/1(q)

== system Masse_MultirotorSimHinf/Sensor Model/Magnetometer/NWU to NED Quaternion2 ==
  qNWU : Inport
  Multiply : Product  Inputs=**
  Quaternion gain : Constant  Value=[1; 1; -1; -1]
  qNED : Outport
  wires:
  Quaternion gain/1 -> Multiply/2
  Multiply/1 -> qNED/1
  qNWU/1 -> Multiply/1

== system Masse_MultirotorSimHinf/Sensor Model/Magnetometer/Quaternion to Rotation Matrix1 ==
  quaternion : Inport
  MATLAB Function : MATLAB Function  TreatAsAtomicUnit=on
  rotationMatrix : Outport
  wires:
  MATLAB Function/1(R) -> rotationMatrix/1
  quaternion/1 -> MATLAB Function/1(q)

== system Masse_MultirotorSimHinf/Sensor Model/Mocap System/NWU to NED Position ==
  posNWU : Inport
  Multiply : Product  Inputs=**
  Position gain : Constant  Value=[1; -1; -1]
  posNED : Outport
  wires:
  posNWU/1 -> Multiply/1
  Multiply/1 -> posNED/1
  Position gain/1 -> Multiply/2

== matlab function Masse_MultirotorSimHinf/Quadrotor Quaternion Model/Equations of motion ==
  data: VBody input; VBodyDot output; nuBody input; Q input; TBody input size=3; tauBody input size=3; F_D input size=3; M_D input size=3; time input; nuBodyDot output; Uav parameter; xiDDot output; Simulation parameter
function [VBodyDot, nuBodyDot, xiDDot] = QuadrotorQuaternionModel(...
    VBody, nuBody, Q, TBody, tauBody, F_D, M_D, time, Uav, Simulation)
%#codegen

%% Handle 2D pitch test
if Uav.PITCH_ONLY
    tauBody = [0; 1; 0] .* tauBody;
    M_D = [0; 1; 0] .* M_D;
end

if ( time < Simulation.T_START_STEP )
    tauBody = [0; 0; 0] .* tauBody;
    M_D = [0; 0; 0] .* M_D;
end

%% Moments and Forces
% Body frame accelerations
VBodyDot  = (1/Uav.M) * (Q'*Uav.G + TBody - cross(nuBody, Uav.M*VBody) + F_D);
nuBodyDot = Uav.I \ (tauBody - cross(nuBody, Uav.I*nuBody) + M_D);

% Inertial frame accelerations
xiDDot = (1/Uav.M)*(Uav.G + Q*(TBody + F_D));
% etaDDot = WInvertDot*nuBody + WInvert*nuBodyDot;

% Check centripetal force in inertial frame
% F_C = R*cross(nuBody,m*VBody);

if Uav.PITCH_ONLY
    xiDDot = [1; 1; 0] .* xiDDot;
end

end

== matlab function Masse_MultirotorSimHinf/Compute Sph ==
  data: V_appBody input; azimuth output; elevation output; radius output
function [azimuth, elevation, radius] = computeSph(V_appBody)
%#codegen

% Convert from polar to spherical coordinates
[ azimuth, elevation, radius ] = cart2sph( V_appBody(1), V_appBody(2), V_appBody(3) );

== matlab function Masse_MultirotorSimHinf/att_controller_ff ==
  data: Textra input; thrustDes output [0..1]; V_appBody input size=3; q input; omega input; Motor parameter; Uav parameter; Aero parameter
function thrustDes  = ffThrust( Textra, V_appBody, q, omega, Motor, Uav, Aero )
%#codegen
    [ azimuth, elevation, windSpeed ] = cart2sph( V_appBody(1), V_appBody(2), V_appBody(3) );
    
    R = QuatToRot(q);
    Rz = R(:,3);
    vertical = [0; 0; 1];
    
    alpha = atan2( norm(cross( Rz, vertical )), dot( Rz, vertical ) );

    if strcmp( Aero.Type, 'Body oriented' )
        U = windSpeed;
        lambda = mean(omega .* Uav.D_PROP / ( 2 * U ));
        
        Cz1 = dot( Aero.Cz1.coefs, [sin(alpha), 1] );
        fz_lift = 0.5 .* Uav.RHO_AIR .* U^2 .* Cz1 * Uav.A_UAV;

        Cz2 = dot( Aero.Cz2.coefs, [alpha, 1]);
        p = Aero.Cz3.coefs;
        Cz3 = p(1) * sin(alpha) + p(2) * ( 1 - exp(-p(3).*lambda) ) .* sin(3*alpha) + ...
            p(4);
        a = 0.5 .* Uav.RHO_AIR .* Cz2 .* Uav.D_PROP^2 .* Uav.A_PROP; % Rotor thrust
        b = 0.5 .* Uav.RHO_AIR .* Cz3 .* U .* Uav.D_PROP .* Uav.A_PROP; % Rotor thrust correction
        
        mg = -Uav.G(3);
        Trequired = ((mg / cos(alpha)) - (fz_lift) + Textra)/4;
        c = Trequired;
        
        omegaRefDes = (-b + sqrt(b^2 + 4*a*c) )/(2*a);
    else
        % Thrust
        x1 = sin(-elevation);
        x2 = windSpeed;
        CT1 = 0.5 * Uav.RHO_AIR * dot( Aero.CT1.coefs, [ 1, x1, x2, x1*x2, x1^2, x2^2, x1^2*x2^2  ] );
        CT2 = 0.5 * Uav.RHO_AIR * dot( Aero.CT2.coefs, [ 1, x1, x2, x1*x2, x1^2, x2^2, x1^2*x2^2  ] );

        % Drag
        x1 = cos(-elevation);
        x2 = mean(omega);
        Cd1 = dot( Aero.Cd1.coefs, [ 1, x1, x2, x1*x2, x1^2, x2^2, x1^2*x2^2  ] );
        Cd2 = dot( Aero.Cd2.coefs, [ 1, x1, x2, x1*x2, x1^2, x2^2, x1^2*x2^2  ] );
        f_D = 0.5 * Uav.RHO_AIR * Cd1 * windSpeed^2 + ...
        0.5 * Uav.RHO_AIR * Cd2 * windSpeed;

        % Lift
        x1 = -elevation;
        x2 = 0;
        Cl = dot( Aero.Cl.coefs, [ 1, x1, x2, x1*x2, x1^2, x2^2, x1^2*x2^2  ] );
        f_l = 0.5 * Uav.RHO_AIR * Cl * windSpeed^2;

        F_D = zeros(3,1);
        F_l = zeros(3,1);
        [ F_D(1), F_D(2), F_D(3) ] = sph2cart( azimuth, elevation, f_D );
        [ F_l(1), F_l(2), F_l(3) ] = sph2cart( azimuth, elevation + pi/2, f_l );

        mg = -Uav.G(3);
        Trequired = mg / cos(alpha) - (F_l(3) + F_D(3)) + Textra;

        omegaRefDes = (-CT2 + sqrt(CT2^2 + 4*CT1*Trequired) )/(2*CT1);
    end


    omegaDes = omegaRefDes; %- mean(omegaDot)*7.006512e-02;
    pwmDes = ( omegaDes/0.84 + 6.528579e2) / 7.969173e-1;

    thrustDes = (pwmDes - 1000) / 1000;
end

function R = QuatToRot( q )
% QUATERNIONTOROTATIONMATRIXMAT Convert quaternion to rotation matrix
% Written by: J.X.J. Bannwarth, 27/03/17
    W = q(1);
    X = q(2);
    Y = q(3);
    Z = q(4);
    
    xx = X * X;
    xy = X * Y;
    xz = X * Z;
    xw = X * W;

    yy = Y * Y;
    yz = Y * Z;
    yw = Y * W;
    
    zz = Z * Z;
    zw = Z * W;

    m00 = 1 - 2 * ( yy + zz );
    m01 =     2 * ( xy - zw );
    m02 =     2 * ( xz + yw );

    m10 =     2 * ( xy + zw );
    m11 = 1 - 2 * ( xx + zz );
    m12 =     2 * ( yz - xw );

    m20 =     2 * ( xz - yw );
    m21 =     2 * ( yz + xw );
    m22 = 1 - 2 * ( xx + yy );
    
    R = [m00 m01 m02;
         m10 m11 m12;
         m20 m21 m22];
    
end

== matlab function Masse_MultirotorSimHinf/Applied wind speed/Relative velocity ==
  data: nuBody input; Uav parameter; VMotorRelBody output size=[3,Uav.N_ROTORS]
function VMotorRelBody = relativeMotorVelocity( nuBody , Uav )
%#codegen
    VMotorRelBody = cross( nuBody, Uav.L_VEC );
end

== matlab function Masse_MultirotorSimHinf/Applied wind speed/Compute V_app2 ==
  data: Q input; UBody output; U input size=3
function UBody = computeUBody(Q, U)
%#codegen

% Rotation matrix from Wind frame to Inertial frame
% Wind frame SEU, inertial frame NED
R_U = [1,  0, 0;
       0, -1, 0;
       0,  0, 1];
   
UBody = Q' * R_U * U;

== matlab function Masse_MultirotorSimHinf/MATLAB Function ==
  data: psi input; R_star_bi output
function R_star_bi = rotation_input(psi)

psi = psi;

R_star_bi = [ 1,  0       , 0       , 0 ;
              0,  cos(psi), sin(psi), 0 ;
              0, -sin(psi), cos(psi), 0 ;
              0,  0       , 0       , 1 ];
          
% sPhi   = sin(eta(1));
% sTheta = sin(eta(2));
% sPsi   = sin(eta(3));
% cPhi   = cos(eta(1));
% cTheta = cos(eta(2));
% cPsi   = cos(eta(3));
% tTheta = tan(eta(2));
% 
% % Body frame to inertial frame
% R = [cPsi*cTheta, cPsi*sTheta*sPhi-sPsi*cPhi, cPsi*sTheta*cPhi+sPsi*sPhi;
%      sPsi*cTheta, sPsi*sTheta*sPhi+cPsi*cPhi, sPsi*sTheta*cPhi-cPsi*sPhi;
%      -sTheta,     cTheta*sPhi,                cTheta*cPhi+sPsi*sPhi];
% R_star_bi = [ 1 0 0 0; [1;0;0] R ];
end

== matlab function Masse_MultirotorSimHinf/Quadrotor Euler Model/Equations of motion ==
  data: VBody input; VBodyDot output; nuBody input; eta input; etaDot input; TBody input size=3; tauBody input size=3; F_D input size=3; M_D input size=3; nuBodyDot output; Uav parameter; xiDDot output; etaDDot output
function [VBodyDot, nuBodyDot, xiDDot, etaDDot] = QuadrotorQuaternionModel(...
    VBody, nuBody, eta, etaDot, TBody, tauBody, F_D, M_D, Uav )
%#codegen

%% Rotation matrices
% Precompute sines and cosines
sPhi   = sin(eta(1));
sTheta = sin(eta(2));
sPsi   = sin(eta(3));
cPhi   = cos(eta(1));
cTheta = cos(eta(2));
cPsi   = cos(eta(3));
tTheta = tan(eta(2));

phiDot   = etaDot(1);
thetaDot = etaDot(2);

% Body frame to inertial frame
R = [cPsi*cTheta, cPsi*sTheta*sPhi-sPsi*cPhi, cPsi*sTheta*cPhi+sPsi*sPhi;
     sPsi*cTheta, sPsi*sTheta*sPhi+cPsi*cPhi, sPsi*sTheta*cPhi-cPsi*sPhi;
     -sTheta,     cTheta*sPhi,                cTheta*cPhi+sPsi*sPhi];

WInvertDot = [...
    0,  phiDot*cPhi*tTheta+thetaDot*sPhi/cTheta^2,    -phiDot*sPhi*cTheta+thetaDot*cPhi/cTheta^2;
    0, -phiDot*sPhi,                                  -phiDot*cPhi;
	0,  phiDot*cPhi/cTheta+phiDot*sPhi*tTheta/cTheta, -phiDot*sPhi/cTheta+thetaDot*cPhi*tTheta/cTheta];

WInvert = [1, sPhi*tTheta,  cPhi*tTheta;
           0, cPhi,        -sPhi;
           0, sPhi/cTheta,  cPhi/cTheta];


%% Moments and Forces
% Body frame accelerations
VBodyDot  = (1/Uav.M) * (R'*Uav.G + TBody - cross(nuBody, Uav.M*VBody) + F_D);
nuBodyDot = Uav.I \ (tauBody - cross(nuBody, Uav.I*nuBody) + M_D);

% Inertial frame accelerations
xiDDot = (1/Uav.M)*(Uav.G + R*TBody + R*F_D);
etaDDot = WInvertDot*nuBody + WInvert*nuBodyDot;

end

== matlab function Masse_MultirotorSimHinf/MATLAB Function1 ==
  data: psi input; R_star_bi output
function R_star_bi = rotation_input(psi)

psi = psi;

R_star_bi = [ 1, 0       ,  0       , 0 ;
              0, cos(psi), -sin(psi), 0 ;
              0, sin(psi),  cos(psi), 0 ;
              0, 0       ,  0       , 1 ];
end

== matlab function Masse_MultirotorSimHinf/Quadrotor Quaternion Model/Normalise Quaternion/MATLAB Function ==
  data: q input; qOut output
function qOut = NormaliseQuat( q )
%NORMALISEQUAT Normalise quaternion
%   Based on PX4 Firmware code: https://github.com/PX4/Firmware
%   Written by:    J.X.J. Bannwarth, 2018/12/11
%   Last modified: J.X.J. Bannwarth, 2018/12/11

    qOut = zeros(4,1);
    normVal = sqrt( dot( q, q ) );
    if normVal ~= 0
        qOut = q ./ normVal;
    end
end

== matlab function Masse_MultirotorSimHinf/Sensor Model/Accelerometer/Quaternion to Rotation Matrix/MATLAB Function ==
  data: q input; R output
function R = QuatToRot( q )
%QUATTOROT Convert quaternion to rotation matrix
%   Written by:    J.X.J. Bannwarth, 2017/03/27
%   Last modified: J.X.J. Bannwarth, 2018/12/11
    W = q(1);
    X = q(2);
    Y = q(3);
    Z = q(4);
    
    xx = X * X;
    xy = X * Y;
    xz = X * Z;
    xw = X * W;

    yy = Y * Y;
    yz = Y * Z;
    yw = Y * W;
    
    zz = Z * Z;
    zw = Z * W;

    m00 = 1 - 2 * ( yy + zz );
    m01 =     2 * ( xy - zw );
    m02 =     2 * ( xz + yw );

    m10 =     2 * ( xy + zw );
    m11 = 1 - 2 * ( xx + zz );
    m12 =     2 * ( yz - xw );

    m20 =     2 * ( xz - yw );
    m21 =     2 * ( yz + xw );
    m22 = 1 - 2 * ( xx + yy );
    
    R = [m00 m01 m02;
         m10 m11 m12;
         m20 m21 m22];   
end

== matlab function Masse_MultirotorSimHinf/Quadrotor Euler Model/Euler Angles to Quaternion/MATLAB Function ==
  data: eulerAngles input; quat output
function quat   = EulerToQuaternion( eulerAngles )
%EULERTOQUATERNION Convert Euler angles to a quaternion
%   Based on PX4 Firmware code: https://github.com/PX4/Firmware
%   Written by: J.X.J. Bannwarth
%   Last modified: 29/08/2016

    roll  = eulerAngles(1);
    pitch = eulerAngles(2);
    yaw   = eulerAngles(3);

    cosPhi_2   = cos(roll / 2.0);
    sinPhi_2   = sin(roll / 2.0);
    cosTheta_2 = cos(pitch / 2.0);
    sinTheta_2 = sin(pitch / 2.0);
    cosPsi_2   = cos(yaw / 2.0);
    sinPsi_2   = sin(yaw / 2.0);

    quat = [ cosPhi_2 .* cosTheta_2 .* cosPsi_2 + sinPhi_2 .* sinTheta_2 .* sinPsi_2;
             sinPhi_2 .* cosTheta_2 .* cosPsi_2 - cosPhi_2 .* sinTheta_2 .* sinPsi_2;
             cosPhi_2 .* sinTheta_2 .* cosPsi_2 + sinPhi_2 .* cosTheta_2 .* sinPsi_2;
             cosPhi_2 .* cosTheta_2 .* sinPsi_2 - sinPhi_2 .* sinTheta_2 .* cosPsi_2 ];

end

== matlab function Masse_MultirotorSimHinf/Quadrotor Euler Model/Compute etaDot ==
  data: nuBody input; eta input; etaDot output
function etaDot = computeEtaDot(nuBody, eta)
%#codegen

sPhi = sin(eta(1));
cPhi = cos(eta(1));
cTheta = cos(eta(2));
tTheta = tan(eta(2));
      
WInverse = [1, sPhi*tTheta,  cPhi*tTheta;
            0, cPhi,        -sPhi;
            0, sPhi/cTheta,  cPhi/cTheta];

etaDot = WInverse*nuBody;

== matlab function Masse_MultirotorSimHinf/Sensor Model/Quaternion to Euler Angles1/MATLAB Function ==
  data: quat input; eul output
function eul   = QuaternionToEuler( quat )
%QUATERNIONTOEULER Convert quaternion to euler angles
%   Based on PX4 Firmware code: https://github.com/PX4/Firmware
%   Written by:    J.X.J. Bannwarth, 2016/08/29
%   Last modified: J.X.J. Bannwarth, 2018/12/11

    eul = [ atan2(2.0 .* (quat(1) .* quat(2) + quat(3) .* quat(4)), ...
                1.0 - 2.0 .* (quat(2) .* quat(2) + quat(3) .* quat(3)));
	        asin(2.0 .* (quat(1) .* quat(3) - quat(4) .* quat(2)));
            atan2(2.0 .* (quat(1) .* quat(4) + quat(2) .* quat(3)), ...
                1.0 - 2.0 .* (quat(3) .* quat(3) + quat(4) .* quat(4))) ];
end

== matlab function Masse_MultirotorSimHinf/Quadrotor Euler Model/compute VBody ==
  data: eta input; VBody output; xiDot input
function VBody = computeVBody(eta, xiDot)
%#codegen

sphi = sin(eta(1));
sTheta = sin(eta(2));
sPsi = sin(eta(3));
cPhi = cos(eta(1));
cTheta = cos(eta(2));
cPsi = cos(eta(3));

R = [ cPsi*cTheta, cPsi*sTheta*sphi-sPsi*cPhi, cPsi*sTheta*cPhi+sPsi*sphi;
	  sPsi*cTheta, sPsi*sTheta*sphi+cPsi*cPhi, sPsi*sTheta*cPhi-cPsi*sphi;
     -sTheta,      cTheta*sphi,                cTheta*cPhi+sPsi*sphi];

VBody = R'*xiDot;

== matlab function Masse_MultirotorSimHinf/att_mixerInput/Euler Angles to Quaternion/MATLAB Function ==
  data: eulerAngles input; quat output
function quat   = EulerToQuaternion( eulerAngles )
%EULERTOQUATERNION Convert Euler angles to a quaternion
%   Based on PX4 Firmware code: https://github.com/PX4/Firmware
%   Written by: J.X.J. Bannwarth
%   Last modified: 29/08/2016

    roll  = eulerAngles(1);
    pitch = eulerAngles(2);
    yaw   = eulerAngles(3);

    cosPhi_2   = cos(roll / 2.0);
    sinPhi_2   = sin(roll / 2.0);
    cosTheta_2 = cos(pitch / 2.0);
    sinTheta_2 = sin(pitch / 2.0);
    cosPsi_2   = cos(yaw / 2.0);
    sinPsi_2   = sin(yaw / 2.0);

    quat = [ cosPhi_2 .* cosTheta_2 .* cosPsi_2 + sinPhi_2 .* sinTheta_2 .* sinPsi_2;
             sinPhi_2 .* cosTheta_2 .* cosPsi_2 - cosPhi_2 .* sinTheta_2 .* sinPsi_2;
             cosPhi_2 .* sinTheta_2 .* cosPsi_2 + sinPhi_2 .* cosTheta_2 .* sinPsi_2;
             cosPhi_2 .* cosTheta_2 .* sinPsi_2 - sinPhi_2 .* sinTheta_2 .* cosPsi_2 ];

end

== matlab function Masse_MultirotorSimHinf/Sensor Model/local_position_estimator/Input assignment ==
  data: armed_armed input; att_q input; mocap_timestamp input; mocap_updated input; mocap_x input; mocap_y input; mocap_z input; sensor_accelerometer_m_s2 input; sensor_baro_alt_meter input; sensor_baro_timestamp_relative input; sensor_timestamp input; sensor_updated input; selfVecIn input; selfVec output
function selfVec = InputAssignment( ...
	                             armed_armed, ...
	                                   att_q, ...
	                         mocap_timestamp, ...
	                           mocap_updated, ...
	                                 mocap_x, ...
	                                 mocap_y, ...
	                                 mocap_z, ...
	               sensor_accelerometer_m_s2, ...
	                   sensor_baro_alt_meter, ...
	          sensor_baro_timestamp_relative, ...
	                        sensor_timestamp, ...
	                          sensor_updated, ...
	                               selfVecIn ...
	)
%#codegen

	selfVec = selfVecIn;

	% Variable assignment
	selfVec(518:518) =                              armed_armed;
	selfVec(519:522) =                                    att_q;
	selfVec(530:530) =                          mocap_timestamp;
	selfVec(531:531) =                            mocap_updated;
	selfVec(532:532) =                                  mocap_x;
	selfVec(533:533) =                                  mocap_y;
	selfVec(534:534) =                                  mocap_z;
	selfVec(537:539) =                sensor_accelerometer_m_s2;
	selfVec(540:540) =                    sensor_baro_alt_meter;
	selfVec(541:541) =           sensor_baro_timestamp_relative;
	selfVec(542:542) =                         sensor_timestamp;
	selfVec(543:543) =                           sensor_updated;
end

== matlab function Masse_MultirotorSimHinf/Sensor Model/local_position_estimator/Output selection ==
  data: est_status_covariances output; est_status_health_flags output; est_status_states output; gpos_vel_n output; gpos_vel_e output; selfVec input; gpos_vel_d output; lpos_vx output; lpos_vy output; lpos_vz output; lpos_x output; lpos_y output; lpos_z output; lpos_yaw output
function [ ...
                   est_status_covariances, ...
                  est_status_health_flags, ...
                        est_status_states, ...
                               gpos_vel_n, ...
                               gpos_vel_e, ...
                               gpos_vel_d, ...
                                  lpos_vx, ...
                                  lpos_vy, ...
                                  lpos_vz, ...
                                   lpos_x, ...
                                   lpos_y, ...
                                   lpos_z, ...
                                 lpos_yaw] ...
   = OutputSelection( selfVec )
%#codegen

	% Variable assignment
	                  est_status_covariances = selfVec(439:448);
	                 est_status_health_flags = selfVec(449:449);
	                       est_status_states = selfVec(454:463);
	                              gpos_vel_n = selfVec(480:480);
	                              gpos_vel_e = selfVec(481:481);
	                              gpos_vel_d = selfVec(482:482);
	                                 lpos_vx = selfVec(501:501);
	                                 lpos_vy = selfVec(502:502);
	                                 lpos_vz = selfVec(503:503);
	                                  lpos_x = selfVec(504:504);
	                                  lpos_y = selfVec(507:507);
	                                  lpos_z = selfVec(508:508);
	                                lpos_yaw = selfVec(512:512);
end
